simulink model "scenario1"  (R2018a)
settings: Solver=VariableStepAuto  StartTime=0.0  StopTime=10.0  RelTol=1e-3
undefined symbols (not defined in the file or in its folder): sigbuilder_block
libraries: fuzblock x1, simulink x1
settings Model: Creator=Iasonas  LastModifiedBy=Iasonas

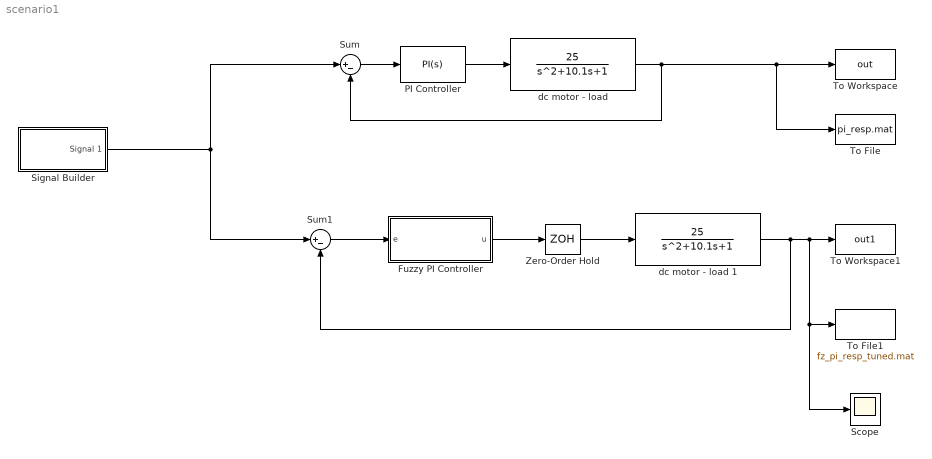
== system scenario1 ==
  Fuzzy PI Controller : Subsystem
  PI Controller : simulink/Continuous/PID Controller  Controller=PI  TimeDomain=Continuous-time  SampleTime=-1  IntegratorMethod=Forward Euler  FilterMethod=Forward Euler  Form=Parallel  UseFilter=on  ControllerParametersSource=internal  P=2.4  I=0.264  D=0  N=100  InitialConditionSource=internal  InitialConditionForIntegrator=0  InitialConditionForFilter=0  ExternalReset=none  LimitOutput=off  UpperSaturationLimit=inf  LowerSaturationLimit=-inf  LinearizeAsGain=on  AntiWindupMode=none  Kb=1  TrackingMode=off  Kt=1  PParamMin=[]  PParamMax=[]  IParamMin=[]  IParamMax=[]  DParamMin=[]  DParamMax=[]  NParamMin=[]  NParamMax=[]  KbParamMin=[]  KbParamMax=[]  KtParamMin=[]  KtParamMax=[]  POutMin=[]  POutMax=[]  IOutMin=[]  IOutMax=[]  DOutMin=[]  DOutMax=[]  NOutMin=[]  NOutMax=[]  KbOutMin=[]  KbOutMax=[]  KtOutMin=[]  KtOutMax=[]  IntegratorOutMin=[]  IntegratorOutMax=[]  FilterOutMin=[]  FilterOutMax=[]  SumOutMin=[]  SumOutMax=[]  SumI1OutMin=[]  SumI1OutMax=[]  SumI2OutMin=[]  SumI2OutMax=[]  SumI3OutMin=[]  SumI3OutMax=[]  SumDOutMin=[]  SumDOutMax=[]  SaturationOutMin=[]  SaturationOutMax=[]  IntegratorContinuousStateAttributes=''  IntegratorStateMustResolveToSignalObject=off  IntegratorRTWStateStorageClass=Auto  FilterContinuousStateAttributes=''  FilterStateMustResolveToSignalObject=off  FilterRTWStateStorageClass=Auto  DifferentiatorICPrevScaledInput=0  DifferentiatorOutMin=[]  DifferentiatorOutMax=[]  FilterDiffOutCoefMin=[]  FilterDiffOutCoefMax=[]  SumDenOutMin=[]  SumDenOutMax=[]  SumNumOutMin=[]  SumNumOutMax=[]  ReciprocalOutMin=[]  ReciprocalOutMax=[]  DivideOutMin=[]  DivideOutMax=[]  TunerSelectOption=Frequency Response Based
  Scope : Scope
  Signal Builder : Subsystem  Tag=STV Subsys  LoadFcn=sigbuilder_block('load');  StartFcn=sigbuilder_block('start');  StopFcn=sigbuilder_block('stop');  ClipboardFcn=sigbuilder_block('clipboard');  mask(Sigbuilder block){tuvar=[0:10]}
      mask help: Simulink:masks:SigbuilderBlock_MD
      mask init:
      | if ~strcmp(get_param(bdroot(gcbh),'SimulationStatus'),'stopped') tuvar = sigbuilder_block('maskInit'); end
      settings: CopyFcn=sigbuilder_block('copy');  DeleteFcn=sigbuilder_block('delete');  ModelCloseFcn=sigbuilder_block('modelClose');  PreSaveFcn=sigbuilder_block('preSave');  PauseFcn=sigbuilder_block('pause');  ContinueFcn=sigbuilder_block('continue');  NameChangeFcn=sigbuilder_block('namechange');  OpenFcn=sigbuilder_block('open',[0 30 1440 722.25 ]);  CloseFcn=sigbuilder_block('close');
      mask Display: plot(0, 0, 100, 100,[2, 2, 32, 32, 2], [68, 8, 8, 68, 68],[32, 2], [38, 38], [32, 19, 2],[53, 60, 44], [32, 17, 17, 2],[16, 16, 31, 31]);txt = getActiveGroup(gcbh);text(2, 100, txt,'verticalAlignment', 'top');
  Sum : Sum  Inputs=|+-
  Sum1 : Sum  Inputs=|+-
  To File : ToFile  Filename=pi_resp.mat  MatrixName=resp  SaveFormat=Timeseries
  To File1 : ToFile  Filename=fz_pi_resp_tuned.mat  MatrixName=resp  SaveFormat=Timeseries
  To Workspace : ToWorkspace  VariableName=out  SaveFormat=Timeseries  SampleTime=-1
  To Workspace1 : ToWorkspace  VariableName=out1  SaveFormat=Timeseries  SampleTime=-1
  Zero-Order Hold : ZeroOrderHold  SampleTime=-1
  "dc motor - load " : TransferFcn  Tag=sadsd  Numerator=[25]  Denominator=[1 10.1 1]
      settings: AttributesFormatString=%<RequirementInfo>
  dc motor - load 1 : TransferFcn  Tag=sadsd  Numerator=[25]  Denominator=[1 10.1 1]
      settings: AttributesFormatString=%<RequirementInfo>
  wires:
  Fuzzy PI Controller/1(u) -> Zero-Order Hold/1
  "dc motor - load "/1 -> Sum/2, To File/1, To Workspace/1
  PI Controller/1 -> "dc motor - load "/1
  Sum1/1 -> Fuzzy PI Controller/1(e)
  Sum/1 -> PI Controller/1
  Signal Builder/1(Signal 1) -> Sum/1, Sum1/1
  dc motor - load 1/1 -> Sum1/2, To File1/1, Scope/1, To Workspace1/1
  Zero-Order Hold/1 -> dc motor - load 1/1

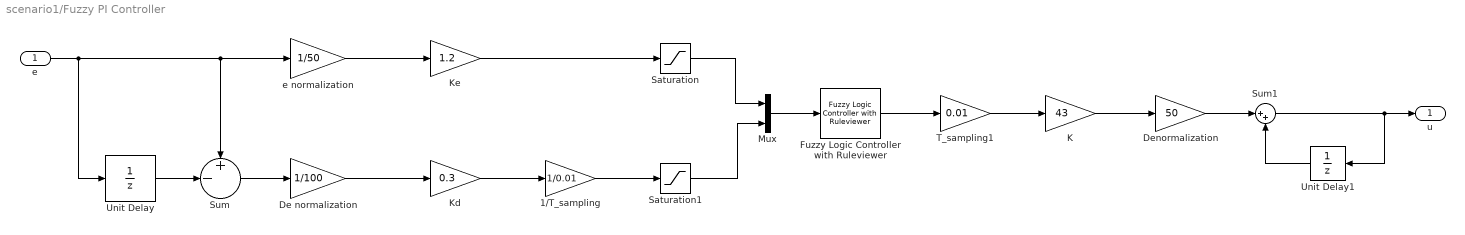
== system scenario1/Fuzzy PI Controller ==
  e : Inport
  1/T_sampling : Gain  Gain=1/0.01
  De normalization : Gain  Gain=1/100
  Denormalization : Gain  Gain=50
  Fuzzy Logic Controller with Ruleviewer : fuzblock/Fuzzy Logic  Controller  with Ruleviewer  fismatrix="readfis(\"FZ_PI.fis\")"  Ts=0.022
  Kd : Gain  Gain=0.3
  Ke : Gain  Gain=1.2
  Mux : Mux  Inputs=2
  Saturation : Saturate  UpperLimit=1  LowerLimit=-1
  Saturation1 : Saturate  UpperLimit=1  LowerLimit=-1
  Sum : Sum  Inputs=+-|
  Sum1 : Sum  Inputs=|++
  T_sampling1 : Gain  Gain=0.01
  Unit Delay : UnitDelay  SampleTime=-1
  Unit Delay1 : UnitDelay  SampleTime=-1
  e normalization : Gain  Gain=1/50
  Κ : Gain  Gain=43
  u : Outport
  wires:
  e/1 -> Unit Delay/1, e normalization/1, Sum/1
  Unit Delay/1 -> Sum/2
  Sum/1 -> De normalization/1
  e normalization/1 -> Ke/1
  De normalization/1 -> Kd/1
  Kd/1 -> 1/T_sampling/1
  Ke/1 -> Saturation/1
  1/T_sampling/1 -> Saturation1/1
  Mux/1 -> Fuzzy Logic Controller with Ruleviewer/1
  Saturation/1 -> Mux/1
  Saturation1/1 -> Mux/2
  Fuzzy Logic Controller with Ruleviewer/1 -> T_sampling1/1
  T_sampling1/1 -> Κ/1
  Κ/1 -> Denormalization/1
  Denormalization/1 -> Sum1/1
  Sum1/1 -> Unit Delay1/1, u/1
  Unit Delay1/1 -> Sum1/2

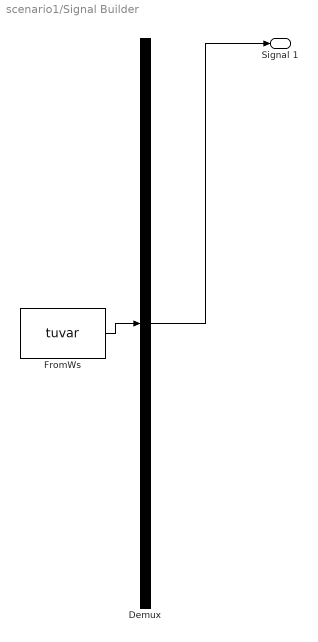
== system scenario1/Signal Builder ==
  Demux : Demux  Tag=STV Demux  Outputs=1
  FromWs : FromWorkspace  Tag=STV FromWs  VariableName=tuvar  SampleTime=0
      SigBuilderData=|
      | common.afterFinalStr = 'Extrapolate'
      | common.sampleTime = 0
      | dataSet.timeRange = [0 20]
      | dataSet.name = 'Group 1'
      | sbobj.Groups.Name = 'Group 1'
      | sbobj.Groups.Signals.Name = 'Signal 1'
      | sbobj.Groups.Signals.XData = [0 5 5 10 10 20]
      | sbobj.Groups.Signals.YData = [50 50 20 20 40 40]
      | sbobj.Groups.TimeRange = [0 20]
  Signal 1 : Outport  Tag=STV Outport
  wires:
  Demux/1 -> Signal 1/1
  FromWs/1 -> Demux/1
